simulink model "Modellezve"  (R2018b)
settings: Solver=VariableStepAuto  StartTime=0.0  StopTime=10.0  RelTol=1e-3
values from neighbouring files (symbols this model uses):
  A = [0 1; 0 -nu/M]    [LQR.m]    (also in LQR_2feladat.m = [0 1 0; 0 0 -omega^2; 0 1 -1/tau]; LQR_sik.m = [0 1 0 0)
  B = [0 ; 1/M]    [LQR.m]    (also in LQR_2feladat.m = [0 omega^2 0]'; LQR_sik.m = [0 0)
  C = [ 1 0]    [LQR.m]    (also in LQR_2feladat.m = [1 0 0]; LQR_sik.m = [1 0 0 0)
  K = R^-1*B'*P    [LQR.m]    (also in LQR_sik.m = inv(R) * B' * P)
  x0 = [-2;20]    [LQR.m]    (also in LQR_2feladat.m = [15, 4, 8]; LQR_sik.m = [100; 20; 50; 20])
settings Model: Creator=brajm  LastModifiedBy=brajm

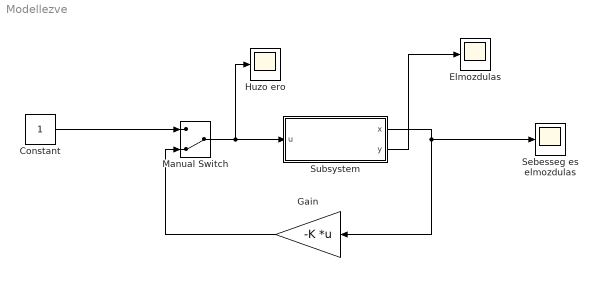
== system Modellezve ==
  Constant : Constant
  Elmozdulas : Scope
  Gain : Gain  Gain=-K  Multiplication=Matrix(K*u)
  Huzo ero : Scope
  Manual Switch : ManualSwitch  CurrentSetting=0
  Sebesseg es elmozdulas : Scope
  Subsystem : Subsystem
  wires:
  Constant/1 -> Manual Switch/1
  Manual Switch/1 -> Huzo ero/1, Subsystem/1(u)
  Subsystem/1(x) -> Gain/1, Sebesseg es elmozdulas/1
  Gain/1 -> Manual Switch/2
  Subsystem/2(y) -> Elmozdulas/1

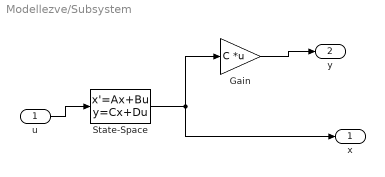
== system Modellezve/Subsystem ==
  u : Inport
  Gain : Gain  Gain=C  Multiplication=Matrix(K*u)
  State-Space : StateSpace  A=A  B=B  C=eye(2)  D=zeros(2,1)  InitialCondition=x0
  x : Outport
  y : Outport  Port=2
  wires:
  u/1 -> State-Space/1
  State-Space/1 -> x/1, Gain/1
  Gain/1 -> y/1
